simulink model "PID_Position_Control"  (R2020a)
settings: Solver=VariableStepAuto  StartTime=0.0  StopTime=10  RelTol=1e-3
undefined symbols (not defined in the file or in its folder): X, Y, Z
libraries: sm_lib x79, nesl_utility x41, simulink x24
(part 2 of 3)

== system PID_Position_Control/PID Control/C9 ==
  Radian : Inport
  Expect : Inport  Port=2
  Discrete Derivative : simulink/Discrete/Discrete Derivative  gainval=1.0  ICPrevScaledInput=0.0  OutMin=[]  OutMax=[]  OutDataType=fixdt(1, 16)  OutScaling=2^-10  DoSatur=off
  Discrete PID Controller : simulink/Continuous/PID Controller  Controller=PID  Form=Parallel  TimeDomain=Discrete-time  UseExternalTs=off  SampleTime=-1  IntegratorMethod=Forward Euler  FilterMethod=Forward Euler  ControllerParametersSource=internal  P=65  I=0.5  D=0.1  UseFilter=on  N=100  TunerSelectOption=Transfer Function Based (PID Tuner App)  InitialConditionSource=internal  InitialConditionForIntegrator=0  InitialConditionForFilter=0  DifferentiatorICPrevScaledInput=0  ExternalReset=none  TrackingMode=off  Kt=1  LimitOutput=off  UpperSaturationLimit=inf  LowerSaturationLimit=-inf  LinearizeAsGain=off  AntiWindupMode=none  Kb=1  POutMin=[]  POutMax=[]  IOutMin=[]  IOutMax=[]  DOutMin=[]  DOutMax=[]  NOutMin=[]  NOutMax=[]  SumOutMin=[]  SumOutMax=[]  SaturationOutMin=[]  SaturationOutMax=[]  PParamMin=[]  PParamMax=[]  IParamMin=[]  IParamMax=[]  DParamMin=[]  DParamMax=[]  NParamMin=[]  NParamMax=[]  KbParamMin=[]  KbParamMax=[]  KtParamMin=[]  KtParamMax=[]  KbOutMin=[]  KbOutMax=[]  KtOutMin=[]  KtOutMax=[]  IntegratorOutMin=[]  IntegratorOutMax=[]  FilterOutMin=[]  FilterOutMax=[]  SumI1OutMin=[]  SumI1OutMax=[]  SumI2OutMin=[]  SumI2OutMax=[]  SumI3OutMin=[]  SumI3OutMax=[]  SumI4OutMin=[]  SumI4OutMax=[]  SumDOutMin=[]  SumDOutMax=[]  DifferentiatorOutMin=[]  DifferentiatorOutMax=[]  FilterDiffOutCoefMin=[]  FilterDiffOutCoefMax=[]  ReciprocalOutMin=[]  ReciprocalOutMax=[]  SumDenOutMin=[]  SumDenOutMax=[]  SumNumOutMin=[]  SumNumOutMax=[]  DivideOutMin=[]  DivideOutMax=[]  UdiffTsProdOutMin=[]  UdiffTsProdOutMax=[]  NTsProdOutMin=[]  NTsProdOutMax=[]  UintegralTsProdOutMin=[]  UintegralTsProdOutMax=[]  UngainTsProdOutMin=[]  UngainTsProdOutMax=[]  IntegratorContinuousStateAttributes=''  IntegratorStateMustResolveToSignalObject=off  IntegratorRTWStateStorageClass=Auto  FilterContinuousStateAttributes=''  FilterStateMustResolveToSignalObject=off  FilterRTWStateStorageClass=Auto  ParallelPVariant=InternalParameters  IdealPVariant=Disabled  IVariant=InternalParameters  DVariant=InternalParameters  IntegratorVariant=Discrete  SatVariant=Disabled  AWVariant=Passthrough  PCopyVariant=Disabled  TRVariant=Disabled  FdbkBlocksVariant=Forward  IdealPFdbkVariant=Disabled  SatFdbkVariant=Disabled  DerivativeFilterVariant=ForwardEulerFilter  NVariant=InternalParameters  NCopyVariant=Disabled  FilterICVariant=InternalICsFilter  IntegratorICVariant=InternalICs  ExternalResetVariant=Disabled  TRSumVariant=Passthrough  SumFdbkVariant=Disabled  SumVariant=Sum_PID  TsampFilterVariant=InternalTs  TsampNgainVariant=Passthrough  TsampIntegralVariant=Passthrough
  Discrete PID Controller1 : simulink/Continuous/PID Controller  Controller=PID  Form=Parallel  TimeDomain=Discrete-time  UseExternalTs=off  SampleTime=-1  IntegratorMethod=Forward Euler  FilterMethod=Forward Euler  ControllerParametersSource=internal  P=27  I=15  D=0.1  UseFilter=on  N=100  TunerSelectOption=Transfer Function Based (PID Tuner App)  InitialConditionSource=internal  InitialConditionForIntegrator=0  InitialConditionForFilter=0  DifferentiatorICPrevScaledInput=0  ExternalReset=none  TrackingMode=off  Kt=1  LimitOutput=off  UpperSaturationLimit=inf  LowerSaturationLimit=-inf  LinearizeAsGain=off  AntiWindupMode=none  Kb=1  POutMin=[]  POutMax=[]  IOutMin=[]  IOutMax=[]  DOutMin=[]  DOutMax=[]  NOutMin=[]  NOutMax=[]  SumOutMin=[]  SumOutMax=[]  SaturationOutMin=[]  SaturationOutMax=[]  PParamMin=[]  PParamMax=[]  IParamMin=[]  IParamMax=[]  DParamMin=[]  DParamMax=[]  NParamMin=[]  NParamMax=[]  KbParamMin=[]  KbParamMax=[]  KtParamMin=[]  KtParamMax=[]  KbOutMin=[]  KbOutMax=[]  KtOutMin=[]  KtOutMax=[]  IntegratorOutMin=[]  IntegratorOutMax=[]  FilterOutMin=[]  FilterOutMax=[]  SumI1OutMin=[]  SumI1OutMax=[]  SumI2OutMin=[]  SumI2OutMax=[]  SumI3OutMin=[]  SumI3OutMax=[]  SumI4OutMin=[]  SumI4OutMax=[]  SumDOutMin=[]  SumDOutMax=[]  DifferentiatorOutMin=[]  DifferentiatorOutMax=[]  FilterDiffOutCoefMin=[]  FilterDiffOutCoefMax=[]  ReciprocalOutMin=[]  ReciprocalOutMax=[]  SumDenOutMin=[]  SumDenOutMax=[]  SumNumOutMin=[]  SumNumOutMax=[]  DivideOutMin=[]  DivideOutMax=[]  UdiffTsProdOutMin=[]  UdiffTsProdOutMax=[]  NTsProdOutMin=[]  NTsProdOutMax=[]  UintegralTsProdOutMin=[]  UintegralTsProdOutMax=[]  UngainTsProdOutMin=[]  UngainTsProdOutMax=[]  IntegratorContinuousStateAttributes=''  IntegratorStateMustResolveToSignalObject=off  IntegratorRTWStateStorageClass=Auto  FilterContinuousStateAttributes=''  FilterStateMustResolveToSignalObject=off  FilterRTWStateStorageClass=Auto  ParallelPVariant=InternalParameters  IdealPVariant=Disabled  IVariant=InternalParameters  DVariant=InternalParameters  IntegratorVariant=Discrete  SatVariant=Disabled  AWVariant=Passthrough  PCopyVariant=Disabled  TRVariant=Disabled  FdbkBlocksVariant=Forward  IdealPFdbkVariant=Disabled  SatFdbkVariant=Disabled  DerivativeFilterVariant=ForwardEulerFilter  NVariant=InternalParameters  NCopyVariant=Disabled  FilterICVariant=InternalICsFilter  IntegratorICVariant=InternalICs  ExternalResetVariant=Disabled  TRSumVariant=Passthrough  SumFdbkVariant=Disabled  SumVariant=Sum_PID  TsampFilterVariant=InternalTs  TsampNgainVariant=Passthrough  TsampIntegralVariant=Passthrough
  Sum : Sum  Inputs=|+-
  Sum1 : Sum  Inputs=|+-
  Tau : Outport  VectorParamsAs1DForOutWhenUnconnected=off
  wires:
  Discrete PID Controller1/1 -> Tau/1
  Sum/1 -> Discrete PID Controller/1
  Radian/1 -> Discrete Derivative/1, Sum/2
  Expect/1 -> Sum/1
  Discrete Derivative/1 -> Sum1/2
  Discrete PID Controller/1 -> Sum1/1
  Sum1/1 -> Discrete PID Controller1/1

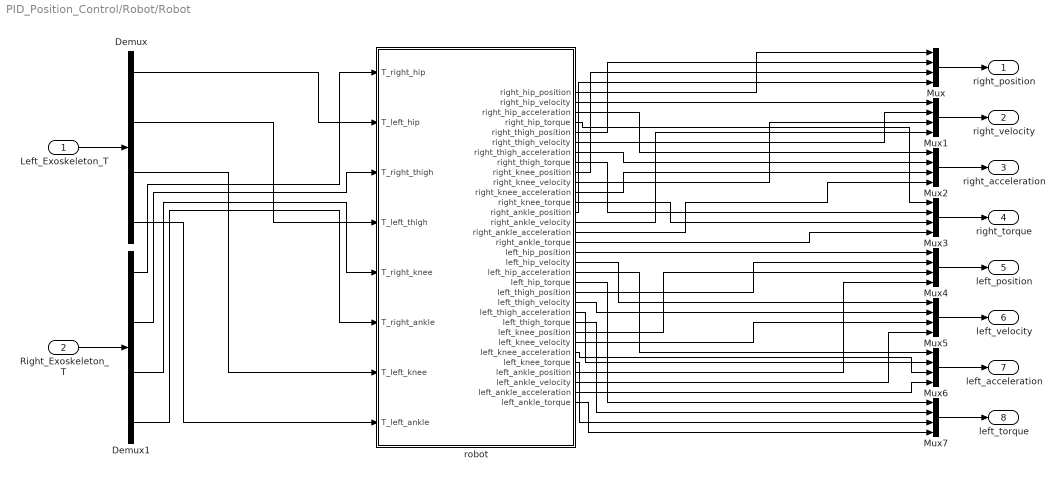
== system PID_Position_Control/Robot/Robot ==
  Left_Exoskeleton_T : Inport
  Right_Exoskeleton_T : Inport  Port=2
  Demux : Demux
  Demux1 : Demux
  Mux{,1..7} (8 alike) : Mux
  robot : Subsystem
  right_position : Outport  VectorParamsAs1DForOutWhenUnconnected=off
  right_velocity : Outport  Port=2  VectorParamsAs1DForOutWhenUnconnected=off
  right_acceleration : Outport  Port=3  VectorParamsAs1DForOutWhenUnconnected=off
  right_torque : Outport  Port=4  VectorParamsAs1DForOutWhenUnconnected=off
  left_position : Outport  Port=5  VectorParamsAs1DForOutWhenUnconnected=off
  left_velocity : Outport  Port=6  VectorParamsAs1DForOutWhenUnconnected=off
  left_acceleration : Outport  Port=7  VectorParamsAs1DForOutWhenUnconnected=off
  left_torque : Outport  Port=8  VectorParamsAs1DForOutWhenUnconnected=off
  wires:
  Demux/1 -> robot/2(T_left_hip)
  robot/14(right_ankle_velocity) -> Mux1/4
  Left_Exoskeleton_T/1 -> Demux/1
  robot/12(right_knee_torque) -> Mux3/3
  robot/31(left_ankle_acceleration) -> Mux6/4
  Demux1/4 -> robot/6(T_right_ankle)
  robot/17(left_hip_position) -> Mux4/1
  robot/22(left_thigh_velocity) -> Mux5/2
  robot/27(left_knee_acceleration) -> Mux6/3
  Mux/1 -> right_position/1
  Mux7/1 -> left_torque/1
  robot/5(right_thigh_position) -> Mux/2
  robot/16(right_ankle_torque) -> Mux3/4
  robot/3(right_hip_acceleration) -> Mux2/1
  robot/18(left_hip_velocity) -> Mux5/1
  Demux1/1 -> robot/1(T_right_hip)
  Demux1/3 -> robot/5(T_right_knee)
  robot/8(right_thigh_torque) -> Mux3/2
  robot/10(right_knee_velocity) -> Mux1/3
  Demux/4 -> robot/8(T_left_ankle)
  robot/24(left_thigh_torque) -> Mux7/2
  Mux3/1 -> right_torque/1
  robot/15(right_ankle_acceleration) -> Mux2/4
  robot/7(right_thigh_acceleration) -> Mux2/2
  robot/21(left_thigh_position) -> Mux4/2
  robot/4(right_hip_torque) -> Mux3/1
  Mux1/1 -> right_velocity/1
  robot/1(right_hip_position) -> Mux/1
  robot/29(left_ankle_position) -> Mux4/4
  robot/20(left_hip_torque) -> Mux7/1
  Mux4/1 -> left_position/1
  robot/25(left_knee_position) -> Mux4/3
  robot/9(right_knee_position) -> Mux/3
  robot/32(left_ankle_torque) -> Mux7/4
  Mux2/1 -> right_acceleration/1
  robot/19(left_hip_acceleration) -> Mux6/1
  Mux5/1 -> left_velocity/1
  robot/11(right_knee_acceleration) -> Mux2/3
  robot/26(left_knee_velocity) -> Mux5/3
  robot/13(right_ankle_position) -> Mux/4
  robot/2(right_hip_velocity) -> Mux1/1
  robot/28(left_knee_torque) -> Mux7/3
  robot/30(left_ankle_velocity) -> Mux5/4
  Mux6/1 -> left_acceleration/1
  Demux/3 -> robot/7(T_left_knee)
  Demux1/2 -> robot/3(T_right_thigh)
  Right_Exoskeleton_T/1 -> Demux1/1
  Demux/2 -> robot/4(T_left_thigh)
  robot/6(right_thigh_velocity) -> Mux1/2
  robot/23(left_thigh_acceleration) -> Mux6/2

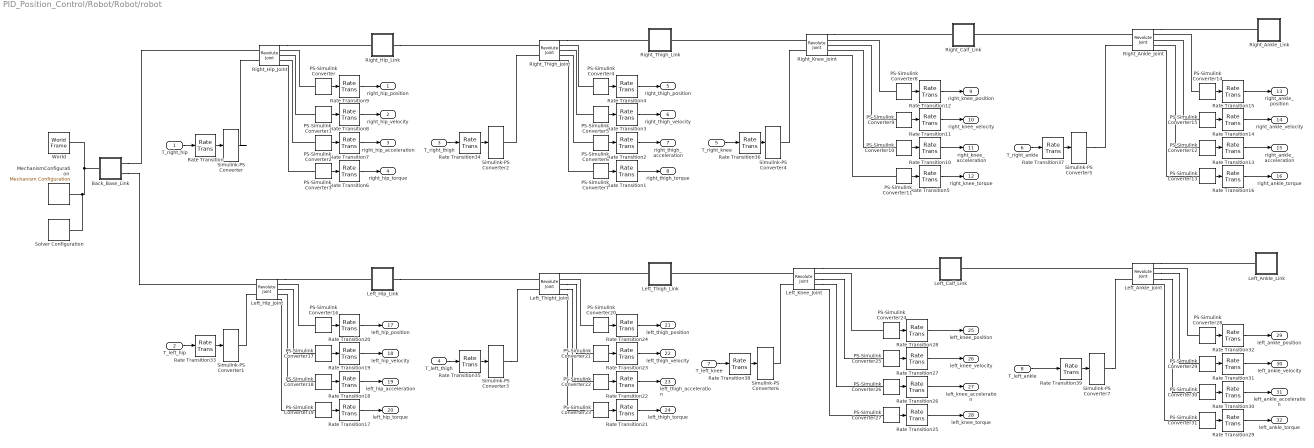
== system PID_Position_Control/Robot/Robot/robot ==
  T_right_hip : Inport
  T_left_hip : Inport  Port=2
  T_right_thigh : Inport  Port=3
  T_left_thigh : Inport  Port=4
  T_right_knee : Inport  Port=5
  T_right_ankle : Inport  Port=6
  T_left_knee : Inport  Port=7
  T_left_ankle : Inport  Port=8
  Back_Base_Link : Subsystem
  Left_Ankle_Joint : sm_lib/Joints/Revolute Joint  JointMode=Normal  SenseConstraintForce=off  SenseConstraintForceX=off  SenseConstraintForceY=off  SenseConstraintForceZ=off  SenseConstraintTorque=off  SenseConstraintTorqueX=off  SenseConstraintTorqueY=off  SenseConstraintTorqueZ=off  SenseTotalForce=off  SenseTotalForceX=off  SenseTotalForceY=off  SenseTotalForceZ=off  SenseTotalTorque=off  SenseTotalTorqueX=off  SenseTotalTorqueY=off  SenseTotalTorqueZ=off  CompositeWrenchDir=FollowerOnBase  CompositeWrenchFrame=BaseFrame  EquilibriumPosition=0  EquilibriumPositionUnits=deg  SpringStiffness=0  SpringStiffnessUnits=N*m/deg  DampingCoefficient=0  DampingCoefficientUnits=m^2*kg/s/rad  TorqueActuationMode=InputTorque  MotionActuationMode=ComputedMotion  SensePosition=on  SenseVelocity=on  SenseAcceleration=on  SenseTorqueForce=on  SenseLowerLimitTorqueForce=off  SenseUpperLimitTorqueForce=off  LowerLimitSpecify=off  LowerLimitBound=0  LowerLimitBoundUnits=rad  LowerLimitStiffness=1e4  LowerLimitStiffnessUnits=N*m/deg  LowerLimitDamping=10  LowerLimitDampingUnits=N*m/(deg/s)  LowerLimitTransitionRegionWidth=0.1  LowerLimitTransitionRegionWidthUnits=deg  UpperLimitSpecify=off  UpperLimitBound=0  UpperLimitBoundUnits=rad  UpperLimitStiffness=1e4  UpperLimitStiffnessUnits=N*m/deg  UpperLimitDamping=10  UpperLimitDampingUnits=N*m/(deg/s)  UpperLimitTransitionRegionWidth=0.1  UpperLimitTransitionRegionWidthUnits=deg  PositionTargetSpecify=off  PositionTargetPriority=High  PositionTargetValue=0  PositionTargetValueUnits=deg  VelocityTargetSpecify=off  VelocityTargetPriority=High  VelocityTargetValue=0  VelocityTargetValueUnits=deg/s
  Left_Ankle_Link : Subsystem
  Left_Calf_Link : Subsystem
  Left_Hip_Joint : sm_lib/Joints/Revolute Joint  JointMode=Normal  SenseConstraintForce=off  SenseConstraintForceX=off  SenseConstraintForceY=off  SenseConstraintForceZ=off  SenseConstraintTorque=off  SenseConstraintTorqueX=off  SenseConstraintTorqueY=off  SenseConstraintTorqueZ=off  SenseTotalForce=off  SenseTotalForceX=off  SenseTotalForceY=off  SenseTotalForceZ=off  SenseTotalTorque=off  SenseTotalTorqueX=off  SenseTotalTorqueY=off  SenseTotalTorqueZ=off  CompositeWrenchDir=FollowerOnBase  CompositeWrenchFrame=BaseFrame  EquilibriumPosition=0  EquilibriumPositionUnits=deg  SpringStiffness=0  SpringStiffnessUnits=N*m/deg  DampingCoefficient=0  DampingCoefficientUnits=m^2*kg/s/rad  TorqueActuationMode=InputTorque  MotionActuationMode=ComputedMotion  SensePosition=on  SenseVelocity=on  SenseAcceleration=on  SenseTorqueForce=on  SenseLowerLimitTorqueForce=off  SenseUpperLimitTorqueForce=off  LowerLimitSpecify=off  LowerLimitBound=0  LowerLimitBoundUnits=rad  LowerLimitStiffness=1e4  LowerLimitStiffnessUnits=N*m/deg  LowerLimitDamping=10  LowerLimitDampingUnits=N*m/(deg/s)  LowerLimitTransitionRegionWidth=0.1  LowerLimitTransitionRegionWidthUnits=deg  UpperLimitSpecify=off  UpperLimitBound=0  UpperLimitBoundUnits=rad  UpperLimitStiffness=1e4  UpperLimitStiffnessUnits=N*m/deg  UpperLimitDamping=10  UpperLimitDampingUnits=N*m/(deg/s)  UpperLimitTransitionRegionWidth=0.1  UpperLimitTransitionRegionWidthUnits=deg  PositionTargetSpecify=off  PositionTargetPriority=High  PositionTargetValue=0  PositionTargetValueUnits=deg  VelocityTargetSpecify=off  VelocityTargetPriority=High  VelocityTargetValue=0  VelocityTargetValueUnits=deg/s
  Left_Hip_Link : Subsystem
  Left_Knee_Joint : sm_lib/Joints/Revolute Joint  JointMode=Normal  SenseConstraintForce=off  SenseConstraintForceX=off  SenseConstraintForceY=off  SenseConstraintForceZ=off  SenseConstraintTorque=off  SenseConstraintTorqueX=off  SenseConstraintTorqueY=off  SenseConstraintTorqueZ=off  SenseTotalForce=off  SenseTotalForceX=off  SenseTotalForceY=off  SenseTotalForceZ=off  SenseTotalTorque=off  SenseTotalTorqueX=off  SenseTotalTorqueY=off  SenseTotalTorqueZ=off  CompositeWrenchDir=FollowerOnBase  CompositeWrenchFrame=BaseFrame  EquilibriumPosition=0  EquilibriumPositionUnits=deg  SpringStiffness=0  SpringStiffnessUnits=N*m/deg  DampingCoefficient=0  DampingCoefficientUnits=m^2*kg/s/rad  TorqueActuationMode=InputTorque  MotionActuationMode=ComputedMotion  SensePosition=on  SenseVelocity=on  SenseAcceleration=on  SenseTorqueForce=on  SenseLowerLimitTorqueForce=off  SenseUpperLimitTorqueForce=off  LowerLimitSpecify=off  LowerLimitBound=0  LowerLimitBoundUnits=rad  LowerLimitStiffness=1e4  LowerLimitStiffnessUnits=N*m/deg  LowerLimitDamping=10  LowerLimitDampingUnits=N*m/(deg/s)  LowerLimitTransitionRegionWidth=0.1  LowerLimitTransitionRegionWidthUnits=deg  UpperLimitSpecify=off  UpperLimitBound=0  UpperLimitBoundUnits=rad  UpperLimitStiffness=1e4  UpperLimitStiffnessUnits=N*m/deg  UpperLimitDamping=10  UpperLimitDampingUnits=N*m/(deg/s)  UpperLimitTransitionRegionWidth=0.1  UpperLimitTransitionRegionWidthUnits=deg  PositionTargetSpecify=off  PositionTargetPriority=High  PositionTargetValue=0  PositionTargetValueUnits=deg  VelocityTargetSpecify=off  VelocityTargetPriority=High  VelocityTargetValue=0  VelocityTargetValueUnits=deg/s
  Left_Thigh_Link : Subsystem
  Left_Thight_Joint : sm_lib/Joints/Revolute Joint  JointMode=Normal  SenseConstraintForce=off  SenseConstraintForceX=off  SenseConstraintForceY=off  SenseConstraintForceZ=off  SenseConstraintTorque=off  SenseConstraintTorqueX=off  SenseConstraintTorqueY=off  SenseConstraintTorqueZ=off  SenseTotalForce=off  SenseTotalForceX=off  SenseTotalForceY=off  SenseTotalForceZ=off  SenseTotalTorque=off  SenseTotalTorqueX=off  SenseTotalTorqueY=off  SenseTotalTorqueZ=off  CompositeWrenchDir=FollowerOnBase  CompositeWrenchFrame=BaseFrame  EquilibriumPosition=0  EquilibriumPositionUnits=deg  SpringStiffness=0  SpringStiffnessUnits=N*m/deg  DampingCoefficient=0  DampingCoefficientUnits=m^2*kg/s/rad  TorqueActuationMode=InputTorque  MotionActuationMode=ComputedMotion  SensePosition=on  SenseVelocity=on  SenseAcceleration=on  SenseTorqueForce=on  SenseLowerLimitTorqueForce=off  SenseUpperLimitTorqueForce=off  LowerLimitSpecify=off  LowerLimitBound=0  LowerLimitBoundUnits=rad  LowerLimitStiffness=1e4  LowerLimitStiffnessUnits=N*m/deg  LowerLimitDamping=10  LowerLimitDampingUnits=N*m/(deg/s)  LowerLimitTransitionRegionWidth=0.1  LowerLimitTransitionRegionWidthUnits=deg  UpperLimitSpecify=off  UpperLimitBound=0  UpperLimitBoundUnits=rad  UpperLimitStiffness=1e4  UpperLimitStiffnessUnits=N*m/deg  UpperLimitDamping=10  UpperLimitDampingUnits=N*m/(deg/s)  UpperLimitTransitionRegionWidth=0.1  UpperLimitTransitionRegionWidthUnits=deg  PositionTargetSpecify=off  PositionTargetPriority=High  PositionTargetValue=0  PositionTargetValueUnits=deg  VelocityTargetSpecify=off  VelocityTargetPriority=High  VelocityTargetValue=0  VelocityTargetValueUnits=deg/s
  MechanismConfiguration : sm_lib/Utilities/Mechanism Configuration  UniformGravity=Constant  GravityVector=[0 0 -9.80665]  GravityUnits=m/s^2  LinearizationDelta=0.001
  PS-Simulink Converter{,4,8,14,16,20,24,28} (8 alike) : nesl_utility/PS-Simulink Converter  PhysicalDomain=network_engine_domain  SubClassName=ps_output  LeftPortType=input  RightPortType=output  PseudoPeriodic=off  Frequencies=[]  Unit=rad  AffineConversion=off
  PS-Simulink Converter{1,5,9,15,17,21,25,29} (8 alike) : nesl_utility/PS-Simulink Converter  PhysicalDomain=network_engine_domain  SubClassName=ps_output  LeftPortType=input  RightPortType=output  PseudoPeriodic=off  Frequencies=[]  Unit=rad/s  AffineConversion=off
  PS-Simulink Converter{2,6,10,12,18,22,26,30} (8 alike) : nesl_utility/PS-Simulink Converter  PhysicalDomain=network_engine_domain  SubClassName=ps_output  LeftPortType=input  RightPortType=output  PseudoPeriodic=off  Frequencies=[]  Unit=1  AffineConversion=off
  PS-Simulink Converter{3,7,11,13,19,23,27,31} (8 alike) : nesl_utility/PS-Simulink Converter  PhysicalDomain=network_engine_domain  SubClassName=ps_output  LeftPortType=input  RightPortType=output  PseudoPeriodic=off  Frequencies=[]  Unit=N*m  AffineConversion=off
  Rate Transition{,1..39} (40 alike) : RateTransition
  Right_Ankle_Joint : sm_lib/Joints/Revolute Joint  JointMode=Normal  SenseConstraintForce=off  SenseConstraintForceX=off  SenseConstraintForceY=off  SenseConstraintForceZ=off  SenseConstraintTorque=off  SenseConstraintTorqueX=off  SenseConstraintTorqueY=off  SenseConstraintTorqueZ=off  SenseTotalForce=off  SenseTotalForceX=off  SenseTotalForceY=off  SenseTotalForceZ=off  SenseTotalTorque=off  SenseTotalTorqueX=off  SenseTotalTorqueY=off  SenseTotalTorqueZ=off  CompositeWrenchDir=FollowerOnBase  CompositeWrenchFrame=BaseFrame  EquilibriumPosition=0  EquilibriumPositionUnits=deg  SpringStiffness=0  SpringStiffnessUnits=N*m/deg  DampingCoefficient=0  DampingCoefficientUnits=m^2*kg/s/rad  TorqueActuationMode=InputTorque  MotionActuationMode=ComputedMotion  SensePosition=on  SenseVelocity=on  SenseAcceleration=on  SenseTorqueForce=on  SenseLowerLimitTorqueForce=off  SenseUpperLimitTorqueForce=off  LowerLimitSpecify=off  LowerLimitBound=0  LowerLimitBoundUnits=rad  LowerLimitStiffness=1e4  LowerLimitStiffnessUnits=N*m/deg  LowerLimitDamping=10  LowerLimitDampingUnits=N*m/(deg/s)  LowerLimitTransitionRegionWidth=0.1  LowerLimitTransitionRegionWidthUnits=deg  UpperLimitSpecify=off  UpperLimitBound=0  UpperLimitBoundUnits=rad  UpperLimitStiffness=1e4  UpperLimitStiffnessUnits=N*m/deg  UpperLimitDamping=10  UpperLimitDampingUnits=N*m/(deg/s)  UpperLimitTransitionRegionWidth=0.1  UpperLimitTransitionRegionWidthUnits=deg  PositionTargetSpecify=off  PositionTargetPriority=High  PositionTargetValue=0  PositionTargetValueUnits=deg  VelocityTargetSpecify=off  VelocityTargetPriority=High  VelocityTargetValue=0  VelocityTargetValueUnits=deg/s
  Right_Ankle_Link : Subsystem
  Right_Calf_Link : Subsystem
  Right_Hip_Joint : sm_lib/Joints/Revolute Joint  JointMode=Normal  SenseConstraintForce=off  SenseConstraintForceX=off  SenseConstraintForceY=off  SenseConstraintForceZ=off  SenseConstraintTorque=off  SenseConstraintTorqueX=off  SenseConstraintTorqueY=off  SenseConstraintTorqueZ=off  SenseTotalForce=off  SenseTotalForceX=off  SenseTotalForceY=off  SenseTotalForceZ=off  SenseTotalTorque=off  SenseTotalTorqueX=off  SenseTotalTorqueY=off  SenseTotalTorqueZ=off  CompositeWrenchDir=FollowerOnBase  CompositeWrenchFrame=BaseFrame  EquilibriumPosition=0  EquilibriumPositionUnits=deg  SpringStiffness=0  SpringStiffnessUnits=N*m/deg  DampingCoefficient=0  DampingCoefficientUnits=m^2*kg/s/rad  TorqueActuationMode=InputTorque  MotionActuationMode=ComputedMotion  SensePosition=on  SenseVelocity=on  SenseAcceleration=on  SenseTorqueForce=on  SenseLowerLimitTorqueForce=off  SenseUpperLimitTorqueForce=off  LowerLimitSpecify=off  LowerLimitBound=0  LowerLimitBoundUnits=rad  LowerLimitStiffness=1e4  LowerLimitStiffnessUnits=N*m/deg  LowerLimitDamping=10  LowerLimitDampingUnits=N*m/(deg/s)  LowerLimitTransitionRegionWidth=0.1  LowerLimitTransitionRegionWidthUnits=deg  UpperLimitSpecify=off  UpperLimitBound=0  UpperLimitBoundUnits=rad  UpperLimitStiffness=1e4  UpperLimitStiffnessUnits=N*m/deg  UpperLimitDamping=10  UpperLimitDampingUnits=N*m/(deg/s)  UpperLimitTransitionRegionWidth=0.1  UpperLimitTransitionRegionWidthUnits=deg  PositionTargetSpecify=off  PositionTargetPriority=High  PositionTargetValue=0  PositionTargetValueUnits=deg  VelocityTargetSpecify=off  VelocityTargetPriority=High  VelocityTargetValue=0  VelocityTargetValueUnits=deg/s
  Right_Hip_Link : Subsystem
  Right_Knee_Joint : sm_lib/Joints/Revolute Joint  JointMode=Normal  SenseConstraintForce=off  SenseConstraintForceX=off  SenseConstraintForceY=off  SenseConstraintForceZ=off  SenseConstraintTorque=off  SenseConstraintTorqueX=off  SenseConstraintTorqueY=off  SenseConstraintTorqueZ=off  SenseTotalForce=off  SenseTotalForceX=off  SenseTotalForceY=off  SenseTotalForceZ=off  SenseTotalTorque=off  SenseTotalTorqueX=off  SenseTotalTorqueY=off  SenseTotalTorqueZ=off  CompositeWrenchDir=FollowerOnBase  CompositeWrenchFrame=BaseFrame  EquilibriumPosition=0  EquilibriumPositionUnits=deg  SpringStiffness=0  SpringStiffnessUnits=N*m/deg  DampingCoefficient=0  DampingCoefficientUnits=m^2*kg/s/rad  TorqueActuationMode=InputTorque  MotionActuationMode=ComputedMotion  SensePosition=on  SenseVelocity=on  SenseAcceleration=on  SenseTorqueForce=on  SenseLowerLimitTorqueForce=off  SenseUpperLimitTorqueForce=off  LowerLimitSpecify=off  LowerLimitBound=0  LowerLimitBoundUnits=rad  LowerLimitStiffness=1e4  LowerLimitStiffnessUnits=N*m/deg  LowerLimitDamping=10  LowerLimitDampingUnits=N*m/(deg/s)  LowerLimitTransitionRegionWidth=0.1  LowerLimitTransitionRegionWidthUnits=deg  UpperLimitSpecify=off  UpperLimitBound=0  UpperLimitBoundUnits=rad  UpperLimitStiffness=1e4  UpperLimitStiffnessUnits=N*m/deg  UpperLimitDamping=10  UpperLimitDampingUnits=N*m/(deg/s)  UpperLimitTransitionRegionWidth=0.1  UpperLimitTransitionRegionWidthUnits=deg  PositionTargetSpecify=off  PositionTargetPriority=High  PositionTargetValue=0  PositionTargetValueUnits=deg  VelocityTargetSpecify=off  VelocityTargetPriority=High  VelocityTargetValue=0  VelocityTargetValueUnits=deg/s
  Right_Thigh_Joint : sm_lib/Joints/Revolute Joint  JointMode=Normal  SenseConstraintForce=off  SenseConstraintForceX=off  SenseConstraintForceY=off  SenseConstraintForceZ=off  SenseConstraintTorque=off  SenseConstraintTorqueX=off  SenseConstraintTorqueY=off  SenseConstraintTorqueZ=off  SenseTotalForce=off  SenseTotalForceX=off  SenseTotalForceY=off  SenseTotalForceZ=off  SenseTotalTorque=off  SenseTotalTorqueX=off  SenseTotalTorqueY=off  SenseTotalTorqueZ=off  CompositeWrenchDir=FollowerOnBase  CompositeWrenchFrame=BaseFrame  EquilibriumPosition=0  EquilibriumPositionUnits=deg  SpringStiffness=0  SpringStiffnessUnits=N*m/deg  DampingCoefficient=0  DampingCoefficientUnits=m^2*kg/s/rad  TorqueActuationMode=InputTorque  MotionActuationMode=ComputedMotion  SensePosition=on  SenseVelocity=on  SenseAcceleration=on  SenseTorqueForce=on  SenseLowerLimitTorqueForce=off  SenseUpperLimitTorqueForce=off  LowerLimitSpecify=off  LowerLimitBound=0  LowerLimitBoundUnits=rad  LowerLimitStiffness=1e4  LowerLimitStiffnessUnits=N*m/deg  LowerLimitDamping=10  LowerLimitDampingUnits=N*m/(deg/s)  LowerLimitTransitionRegionWidth=0.1  LowerLimitTransitionRegionWidthUnits=deg  UpperLimitSpecify=off  UpperLimitBound=0  UpperLimitBoundUnits=rad  UpperLimitStiffness=1e4  UpperLimitStiffnessUnits=N*m/deg  UpperLimitDamping=10  UpperLimitDampingUnits=N*m/(deg/s)  UpperLimitTransitionRegionWidth=0.1  UpperLimitTransitionRegionWidthUnits=deg  PositionTargetSpecify=off  PositionTargetPriority=High  PositionTargetValue=0  PositionTargetValueUnits=deg  VelocityTargetSpecify=off  VelocityTargetPriority=High  VelocityTargetValue=0  VelocityTargetValueUnits=deg/s
  Right_Thigh_Link : Subsystem
  Simulink-PS Converter{,1..7} (8 alike) : nesl_utility/Simulink-PS Converter  PhysicalDomain=network_engine_domain  SubClassName=ps_input  LeftPortType=input  RightPortType=output  PseudoPeriodic=off  Frequencies=[]  NoiseDistribution=none  NoiseParameters=[]  Unit=N*m  AffineConversion=off  FilteringAndDerivatives=zero  SimscapeFilterOrder=1  InputFilterTimeConstant=0.001  UdotUserProvided=2
  Solver Configuration : nesl_utility/Solver Configuration  PhysicalDomain=network_engine_domain  SubClassName=solver  LeftPortType=input  RightPortType=generic  Tones=[]  Harmonics=[]  SimulateNoise=off  Profile=off  UseLocalSampling=off  EnableSwitchedLinearOptims=on  FrequencyDomain=off  UseCCode=off  RelTol=0.001  AbsTol=1e-06  MinStep=1e-09  ToWorkspace=off  RevertToSquareIcSolve=off  NumHomotopyIterations=100  PhasorMode=off  PhasorModeNumHarmonics=1  DoDC=off  ResidualTolerance=1e-09  UseLocalSolver=off  LocalSolverChoice=NE_BACKWARD_EULER_ADVANCER  LocalSolverSampleTime=0.001  DoFixedCost=off  MaxNonlinIter=3  MaxModeIter=2  LinearAlgebra=auto  EquationFormulation=NE_TIME_EF  DelaysMemoryBudget=1024  AutomaticFiltering=on  FilteringTimeConstant=0.001  PartitionStorageMethod=AS_NEEDED  PartitionMemoryBudget=1024  PartitionMethod=ROBUST
  World : sm_lib/Frames and Transforms/World Frame
  right_hip_position : Outport  VectorParamsAs1DForOutWhenUnconnected=off
  right_hip_velocity : Outport  Port=2  VectorParamsAs1DForOutWhenUnconnected=off
  right_hip_acceleration : Outport  Port=3  VectorParamsAs1DForOutWhenUnconnected=off
  right_hip_torque : Outport  Port=4  VectorParamsAs1DForOutWhenUnconnected=off
  right_thigh_position : Outport  Port=5  VectorParamsAs1DForOutWhenUnconnected=off
  right_thigh_velocity : Outport  Port=6  VectorParamsAs1DForOutWhenUnconnected=off
  right_thigh_acceleration : Outport  Port=7  VectorParamsAs1DForOutWhenUnconnected=off
  right_thigh_torque : Outport  Port=8  VectorParamsAs1DForOutWhenUnconnected=off
  right_knee_position : Outport  Port=9  VectorParamsAs1DForOutWhenUnconnected=off
  right_knee_velocity : Outport  Port=10  VectorParamsAs1DForOutWhenUnconnected=off
  right_knee_acceleration : Outport  Port=11  VectorParamsAs1DForOutWhenUnconnected=off
  right_knee_torque : Outport  Port=12  VectorParamsAs1DForOutWhenUnconnected=off
  right_ankle_position : Outport  Port=13  VectorParamsAs1DForOutWhenUnconnected=off
  right_ankle_velocity : Outport  Port=14  VectorParamsAs1DForOutWhenUnconnected=off
  right_ankle_acceleration : Outport  Port=15  VectorParamsAs1DForOutWhenUnconnected=off
  right_ankle_torque : Outport  Port=16  VectorParamsAs1DForOutWhenUnconnected=off
  left_hip_position : Outport  Port=17  VectorParamsAs1DForOutWhenUnconnected=off
  left_hip_velocity : Outport  Port=18  VectorParamsAs1DForOutWhenUnconnected=off
  left_hip_acceleration : Outport  Port=19  VectorParamsAs1DForOutWhenUnconnected=off
  left_hip_torque : Outport  Port=20  VectorParamsAs1DForOutWhenUnconnected=off
  left_thigh_position : Outport  Port=21  VectorParamsAs1DForOutWhenUnconnected=off
  left_thigh_velocity : Outport  Port=22  VectorParamsAs1DForOutWhenUnconnected=off
  left_thigh_acceleration : Outport  Port=23  VectorParamsAs1DForOutWhenUnconnected=off
  left_thigh_torque : Outport  Port=24  VectorParamsAs1DForOutWhenUnconnected=off
  left_knee_position : Outport  Port=25  VectorParamsAs1DForOutWhenUnconnected=off
  left_knee_velocity : Outport  Port=26  VectorParamsAs1DForOutWhenUnconnected=off
  left_knee_acceleration : Outport  Port=27  VectorParamsAs1DForOutWhenUnconnected=off
  left_knee_torque : Outport  Port=28  VectorParamsAs1DForOutWhenUnconnected=off
  left_ankle_position : Outport  Port=29  VectorParamsAs1DForOutWhenUnconnected=off
  left_ankle_velocity : Outport  Port=30  VectorParamsAs1DForOutWhenUnconnected=off
  left_ankle_acceleration : Outport  Port=31  VectorParamsAs1DForOutWhenUnconnected=off
  left_ankle_torque : Outport  Port=32  VectorParamsAs1DForOutWhenUnconnected=off
  wires:
  PS-Simulink Converter8/1 -> Rate Transition12/1
  Rate Transition12/1 -> right_knee_position/1
  PS-Simulink Converter9/1 -> Rate Transition11/1
  Rate Transition5/1 -> right_knee_torque/1
  Rate Transition10/1 -> right_knee_acceleration/1
  PS-Simulink Converter3/1 -> Rate Transition6/1
  Rate Transition11/1 -> right_knee_velocity/1
  Rate Transition4/1 -> right_thigh_position/1
  Rate Transition3/1 -> right_thigh_velocity/1
  Rate Transition2/1 -> right_thigh_acceleration/1
  PS-Simulink Converter6/1 -> Rate Transition2/1
  PS-Simulink Converter5/1 -> Rate Transition3/1
  PS-Simulink Converter4/1 -> Rate Transition4/1
  Rate Transition1/1 -> right_thigh_torque/1
  T_right_ankle/1 -> Rate Transition37/1
  Rate Transition37/1 -> Simulink-PS Converter5/1
  Rate Transition39/1 -> Simulink-PS Converter7/1
  Rate Transition35/1 -> Simulink-PS Converter3/1
  T_left_thigh/1 -> Rate Transition35/1
  Rate Transition38/1 -> Simulink-PS Converter6/1
  T_left_knee/1 -> Rate Transition38/1
  T_right_knee/1 -> Rate Transition36/1
  T_right_thigh/1 -> Rate Transition34/1
  Rate Transition8/1 -> right_hip_velocity/1
  Rate Transition7/1 -> right_hip_acceleration/1
  Rate Transition9/1 -> right_hip_position/1
  Rate Transition36/1 -> Simulink-PS Converter4/1
  PS-Simulink Converter16/1 -> Rate Transition20/1
  PS-Simulink Converter19/1 -> Rate Transition17/1
  Rate Transition19/1 -> left_hip_velocity/1
  PS-Simulink Converter17/1 -> Rate Transition19/1
  Rate Transition20/1 -> left_hip_position/1
  Rate Transition18/1 -> left_hip_acceleration/1
  Rate Transition17/1 -> left_hip_torque/1
  T_right_hip/1 -> Rate Transition/1
  Rate Transition34/1 -> Simulink-PS Converter2/1
  PS-Simulink Converter18/1 -> Rate Transition18/1
  PS-Simulink Converter27/1 -> Rate Transition25/1
  Rate Transition25/1 -> left_knee_torque/1
  Rate Transition26/1 -> left_knee_acceleration/1
  Rate Transition28/1 -> left_knee_position/1
  PS-Simulink Converter11/1 -> Rate Transition5/1
  PS-Simulink Converter24/1 -> Rate Transition28/1
  PS-Simulink Converter25/1 -> Rate Transition27/1
  Rate Transition27/1 -> left_knee_velocity/1
  PS-Simulink Converter26/1 -> Rate Transition26/1
  Rate Transition/1 -> Simulink-PS Converter/1
  T_left_ankle/1 -> Rate Transition39/1
  PS-Simulink Converter23/1 -> Rate Transition21/1
  Rate Transition21/1 -> left_thigh_torque/1
  PS-Simulink Converter22/1 -> Rate Transition22/1
  PS-Simulink Converter21/1 -> Rate Transition23/1
  Rate Transition23/1 -> left_thigh_velocity/1
  PS-Simulink Converter1/1 -> Rate Transition8/1
  Rate Transition24/1 -> left_thigh_position/1
  PS-Simulink Converter7/1 -> Rate Transition1/1
  T_left_hip/1 -> Rate Transition33/1
  Rate Transition33/1 -> Simulink-PS Converter1/1
  PS-Simulink Converter12/1 -> Rate Transition13/1
  PS-Simulink Converter13/1 -> Rate Transition16/1
  PS-Simulink Converter2/1 -> Rate Transition7/1
  PS-Simulink Converter10/1 -> Rate Transition10/1
  PS-Simulink Converter/1 -> Rate Transition9/1
  PS-Simulink Converter15/1 -> Rate Transition14/1
  PS-Simulink Converter20/1 -> Rate Transition24/1
  Rate Transition14/1 -> right_ankle_velocity/1
  Rate Transition22/1 -> left_thigh_acceleration/1
  Rate Transition15/1 -> right_ankle_position/1
  PS-Simulink Converter30/1 -> Rate Transition30/1
  Rate Transition31/1 -> left_ankle_velocity/1
  PS-Simulink Converter29/1 -> Rate Transition31/1
  Rate Transition13/1 -> right_ankle_acceleration/1
  Rate Transition6/1 -> right_hip_torque/1
  Rate Transition29/1 -> left_ankle_torque/1
  Rate Transition32/1 -> left_ankle_position/1
  PS-Simulink Converter14/1 -> Rate Transition15/1
  Rate Transition16/1 -> right_ankle_torque/1
  PS-Simulink Converter31/1 -> Rate Transition29/1
  Rate Transition30/1 -> left_ankle_acceleration/1
  PS-Simulink Converter28/1 -> Rate Transition32/1
  connections:
  Back_Base_Link/LConn1 -- World/RConn1 -- Solver Configuration/RConn1 -- MechanismConfiguration/RConn1
  PS-Simulink Converter19/LConn1 -- Left_Hip_Joint/RConn5
  PS-Simulink Converter8/LConn1 -- Right_Knee_Joint/RConn2
  Right_Thigh_Joint/LConn2 -- Simulink-PS Converter2/RConn1
  PS-Simulink Converter10/LConn1 -- Right_Knee_Joint/RConn4
  Simulink-PS Converter7/RConn1 -- Left_Ankle_Joint/LConn2
  PS-Simulink Converter27/LConn1 -- Left_Knee_Joint/RConn5
  PS-Simulink Converter17/LConn1 -- Left_Hip_Joint/RConn3
  Right_Hip_Link/RConn1 -- Right_Thigh_Joint/LConn1
  Simulink-PS Converter5/RConn1 -- Right_Ankle_Joint/LConn2
  PS-Simulink Converter3/LConn1 -- Right_Hip_Joint/RConn5
  PS-Simulink Converter5/LConn1 -- Right_Thigh_Joint/RConn3
  Left_Ankle_Joint/RConn3 -- PS-Simulink Converter29/LConn1
  PS-Simulink Converter/LConn1 -- Right_Hip_Joint/RConn2
  PS-Simulink Converter31/LConn1 -- Left_Ankle_Joint/RConn5
  Right_Ankle_Joint/RConn1 -- Right_Ankle_Link/LConn1
  PS-Simulink Converter18/LConn1 -- Left_Hip_Joint/RConn4
  PS-Simulink Converter23/LConn1 -- Left_Thight_Joint/RConn5
  PS-Simulink Converter2/LConn1 -- Right_Hip_Joint/RConn4
  PS-Simulink Converter7/LConn1 -- Right_Thigh_Joint/RConn5
  Simulink-PS Converter1/RConn1 -- Left_Hip_Joint/LConn2
  Left_Thight_Joint/RConn3 -- PS-Simulink Converter21/LConn1
  Back_Base_Link/RConn2 -- Left_Hip_Joint/LConn1
  Left_Knee_Joint/RConn4 -- PS-Simulink Converter26/LConn1
  Back_Base_Link/RConn1 -- Right_Hip_Joint/LConn1
  PS-Simulink Converter12/LConn1 -- Right_Ankle_Joint/RConn4
  PS-Simulink Converter28/LConn1 -- Left_Ankle_Joint/RConn2
  PS-Simulink Converter14/LConn1 -- Right_Ankle_Joint/RConn2
  PS-Simulink Converter11/LConn1 -- Right_Knee_Joint/RConn5
  Left_Thight_Joint/RConn4 -- PS-Simulink Converter22/LConn1
  PS-Simulink Converter4/LConn1 -- Right_Thigh_Joint/RConn2
  Right_Knee_Joint/LConn2 -- Simulink-PS Converter4/RConn1
  Left_Knee_Joint/RConn3 -- PS-Simulink Converter25/LConn1
  Right_Hip_Joint/RConn1 -- Right_Hip_Link/LConn1
  PS-Simulink Converter16/LConn1 -- Left_Hip_Joint/RConn2
  Left_Ankle_Joint/LConn1 -- Left_Calf_Link/RConn1
  PS-Simulink Converter1/LConn1 -- Right_Hip_Joint/RConn3
  Left_Ankle_Joint/RConn1 -- Left_Ankle_Link/LConn1
  Left_Hip_Joint/RConn1 -- Left_Hip_Link/LConn1
  Left_Knee_Joint/LConn1 -- Left_Thigh_Link/RConn1
  Right_Knee_Joint/LConn1 -- Right_Thigh_Link/RConn1
  Right_Knee_Joint/RConn1 -- Right_Calf_Link/LConn1
  PS-Simulink Converter15/LConn1 -- Right_Ankle_Joint/RConn3
  Left_Hip_Link/RConn1 -- Left_Thight_Joint/LConn1
  Simulink-PS Converter3/RConn1 -- Left_Thight_Joint/LConn2
  Simulink-PS Converter/RConn1 -- Right_Hip_Joint/LConn2
  Right_Thigh_Joint/RConn1 -- Right_Thigh_Link/LConn1
  PS-Simulink Converter24/LConn1 -- Left_Knee_Joint/RConn2
  Left_Thigh_Link/LConn1 -- Left_Thight_Joint/RConn1
  PS-Simulink Converter20/LConn1 -- Left_Thight_Joint/RConn2
  Right_Ankle_Joint/LConn1 -- Right_Calf_Link/RConn1
  Left_Knee_Joint/RConn1 -- Left_Calf_Link/LConn1
  PS-Simulink Converter13/LConn1 -- Right_Ankle_Joint/RConn5
  PS-Simulink Converter9/LConn1 -- Right_Knee_Joint/RConn3
  Left_Ankle_Joint/RConn4 -- PS-Simulink Converter30/LConn1
  PS-Simulink Converter6/LConn1 -- Right_Thigh_Joint/RConn4
  Simulink-PS Converter6/RConn1 -- Left_Knee_Joint/LConn2

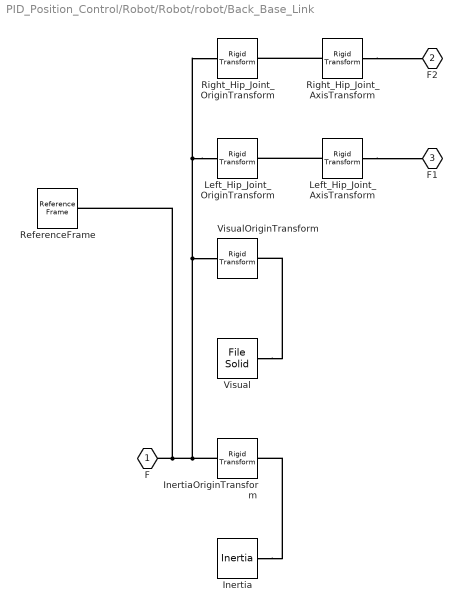
== system PID_Position_Control/Robot/Robot/robot/Back_Base_Link ==
  Inertia : sm_lib/Body Elements/Inertia  InertiaType=Custom  Mass=7.1666344893724  MassUnits=kg  CenterOfMass=[0, 0, 0]  CenterOfMassUnits=m  MomentsOfInertia=[0.287991764742564, 0.218183102338654, 0.12372998211452]  MomentsOfInertiaUnits=kg*m^2  ProductsOfInertia=[-5.72291606644722e-09, 0.00975876307734881, 4.03119244398634e-09]  ProductsOfInertiaUnits=kg*m^2  GraphicType=None  MarkerShape=Inertia  MarkerSize=20  GraphicVisPropType=SimpleVisualProperties  GraphicDiffuseColor=[0.5 0.5 0.5]  GraphicSpecularColor=[0.5 0.5 0.5 1.0]  GraphicAmbientColor=[0.15 0.15 0.15 1.0]  GraphicEmissiveColor=[0.0 0.0 0.0 1.0]  GraphicShininess=75  GraphicOpacity=1.0
  InertiaOriginTransform : sm_lib/Frames and Transforms/Rigid Transform  TranslationMethod=Cartesian  TranslationStandardOffset=0  TranslationLengthUnit=m  TranslationStandardAxis=+Z  TranslationCartesianOffset=[0.102999774541297, 1.05565171604205e-08, -0.01817224156931]  TranslationROffset=0  TranslationROffsetUnits=m  TranslationZOffset=0  TranslationZOffsetUnits=m  TranslationThetaOffset=0  TranslationThetaOffsetUnits=deg  RotationMethod=RotationSequence  RotationAngleUnits=deg  RotationStandardAxis=+Z  RotationAngle=0.0  RotationArbitraryAxis=[0 0 1]  FollAlignAxisA=+X  BaseAlignAxisA=+Y  FollAlignAxisB=+Y  BaseAlignAxisB=+Z  RotationSequenceAxes=BaseAxes  RotationSequence=XYZ  RotationSequenceAngles=[0, 0, 0]  RotationSequenceAnglesUnits=rad  RotationMatrix=[1 0 0; 0 1 0; 0 0 1]
  Left_Hip_Joint_AxisTransform : sm_lib/Frames and Transforms/Rigid Transform  TranslationMethod=Cartesian  TranslationStandardOffset=0  TranslationLengthUnit=m  TranslationStandardAxis=+Z  TranslationCartesianOffset=[0, 0, 0]  TranslationROffset=0  TranslationROffsetUnits=m  TranslationZOffset=0  TranslationZOffsetUnits=m  TranslationThetaOffset=0  TranslationThetaOffsetUnits=deg  RotationMethod=ArbitraryAxis  RotationAngleUnits=rad  RotationStandardAxis=+Z  RotationAngle=3.141592653589793  RotationArbitraryAxis=[1, 0, 0]  FollAlignAxisA=+X  BaseAlignAxisA=+Y  FollAlignAxisB=+Y  BaseAlignAxisB=+Z  RotationSequenceAxes=FollowerAxes  RotationSequence=XYX  RotationSequenceAngles=[0 0 0]  RotationSequenceAnglesUnits=deg  RotationMatrix=[1 0 0; 0 1 0; 0 0 1]
  Left_Hip_Joint_OriginTransform : sm_lib/Frames and Transforms/Rigid Transform  TranslationMethod=Cartesian  TranslationStandardOffset=0  TranslationLengthUnit=m  TranslationStandardAxis=+Z  TranslationCartesianOffset=[0.2243, 0.208, -0.283]  TranslationROffset=0  TranslationROffsetUnits=m  TranslationZOffset=0  TranslationZOffsetUnits=m  TranslationThetaOffset=0  TranslationThetaOffsetUnits=deg  RotationMethod=RotationSequence  RotationAngleUnits=deg  RotationStandardAxis=+Z  RotationAngle=0.0  RotationArbitraryAxis=[0 0 1]  FollAlignAxisA=+X  BaseAlignAxisA=+Y  FollAlignAxisB=+Y  BaseAlignAxisB=+Z  RotationSequenceAxes=BaseAxes  RotationSequence=XYZ  RotationSequenceAngles=[0, 0, 0]  RotationSequenceAnglesUnits=rad  RotationMatrix=[1 0 0; 0 1 0; 0 0 1]
  ReferenceFrame : sm_lib/Frames and Transforms/Reference Frame
  Right_Hip_Joint_AxisTransform : sm_lib/Frames and Transforms/Rigid Transform  TranslationMethod=Cartesian  TranslationStandardOffset=0  TranslationLengthUnit=m  TranslationStandardAxis=+Z  TranslationCartesianOffset=[0, 0, 0]  TranslationROffset=0  TranslationROffsetUnits=m  TranslationZOffset=0  TranslationZOffsetUnits=m  TranslationThetaOffset=0  TranslationThetaOffsetUnits=deg  RotationMethod=ArbitraryAxis  RotationAngleUnits=rad  RotationStandardAxis=+Z  RotationAngle=0  RotationArbitraryAxis=[1, 0, 0]  FollAlignAxisA=+X  BaseAlignAxisA=+Y  FollAlignAxisB=+Y  BaseAlignAxisB=+Z  RotationSequenceAxes=FollowerAxes  RotationSequence=XYX  RotationSequenceAngles=[0 0 0]  RotationSequenceAnglesUnits=deg  RotationMatrix=[1 0 0; 0 1 0; 0 0 1]
  Right_Hip_Joint_OriginTransform : sm_lib/Frames and Transforms/Rigid Transform  TranslationMethod=Cartesian  TranslationStandardOffset=0  TranslationLengthUnit=m  TranslationStandardAxis=+Z  TranslationCartesianOffset=[0.2243, -0.208, -0.283]  TranslationROffset=0  TranslationROffsetUnits=m  TranslationZOffset=0  TranslationZOffsetUnits=m  TranslationThetaOffset=0  TranslationThetaOffsetUnits=deg  RotationMethod=RotationSequence  RotationAngleUnits=deg  RotationStandardAxis=+Z  RotationAngle=0.0  RotationArbitraryAxis=[0 0 1]  FollAlignAxisA=+X  BaseAlignAxisA=+Y  FollAlignAxisB=+Y  BaseAlignAxisB=+Z  RotationSequenceAxes=BaseAxes  RotationSequence=XYZ  RotationSequenceAngles=[0, 0, 0]  RotationSequenceAnglesUnits=rad  RotationMatrix=[1 0 0; 0 1 0; 0 0 1]
  Visual : sm_lib/Body Elements/File Solid  ExtGeomFileName=C:\Users\河明山\Desktop\毕业设计\下肢\meshes\Back_Base_Link.STL  UnitType=Custom  ExtGeomFileUnits=m  StepReaderType=HEX  ExportConvexHullGeometry=off  InertiaType=Custom  Mass=0  MassUnits=kg  CenterOfMass=[0, 0, 0]  CenterOfMassUnits=m  MomentsOfInertia=[0, 0, 0]  MomentsOfInertiaUnits=kg*m^2  ProductsOfInertia=[0, 0, 0]  ProductsOfInertiaUnits=kg*m^2  BasedOnType=DensityFromFile  Density=1000  DensityUnits=kg/m^3  DoExposeReferenceFrame=on  SerializedFrames=<Frames/>  GraphicType=FromGeometry  MarkerShape=Sphere  MarkerSize=10  GraphicVisPropType=SimpleVisualProperties  GraphicDiffuseColor=[0.898039215686275, 0.917647058823529, 0.929411764705882]  GraphicSpecularColor=[0.5 0.5 0.5 1.0]  GraphicAmbientColor=[0.15 0.15 0.15 1.0]  GraphicEmissiveColor=[0.0 0.0 0.0 1.0]  GraphicShininess=75  GraphicOpacity=1
  VisualOriginTransform : sm_lib/Frames and Transforms/Rigid Transform  TranslationMethod=Cartesian  TranslationStandardOffset=0  TranslationLengthUnit=m  TranslationStandardAxis=+Z  TranslationCartesianOffset=[0, 0, 0]  TranslationROffset=0  TranslationROffsetUnits=m  TranslationZOffset=0  TranslationZOffsetUnits=m  TranslationThetaOffset=0  TranslationThetaOffsetUnits=deg  RotationMethod=RotationSequence  RotationAngleUnits=deg  RotationStandardAxis=+Z  RotationAngle=0.0  RotationArbitraryAxis=[0 0 1]  FollAlignAxisA=+X  BaseAlignAxisA=+Y  FollAlignAxisB=+Y  BaseAlignAxisB=+Z  RotationSequenceAxes=BaseAxes  RotationSequence=XYZ  RotationSequenceAngles=[0, 0, 0]  RotationSequenceAnglesUnits=rad  RotationMatrix=[1 0 0; 0 1 0; 0 0 1]
  F : PMIOPort  Side=Left
  F2 : PMIOPort  Port=2  Side=Right
  F1 : PMIOPort  Port=3  Side=Right
  connections:
  Inertia/RConn1 -- InertiaOriginTransform/RConn1
  Left_Hip_Joint_AxisTransform/RConn1 -- F1/RConn1
  Left_Hip_Joint_AxisTransform/LConn1 -- Left_Hip_Joint_OriginTransform/RConn1
  Left_Hip_Joint_OriginTransform/LConn1 -- InertiaOriginTransform/LConn1 -- ReferenceFrame/RConn1 -- F/RConn1 -- VisualOriginTransform/LConn1 -- Right_Hip_Joint_OriginTransform/LConn1
  Right_Hip_Joint_AxisTransform/RConn1 -- F2/RConn1
  Right_Hip_Joint_AxisTransform/LConn1 -- Right_Hip_Joint_OriginTransform/RConn1
  Visual/RConn1 -- VisualOriginTransform/RConn1

== system PID_Position_Control/Robot/Robot/robot/Left_Ankle_Link ==
  Inertia : sm_lib/Body Elements/Inertia  InertiaType=Custom  Mass=1.19036450922831  MassUnits=kg  CenterOfMass=[0, 0, 0]  CenterOfMassUnits=m  MomentsOfInertia=[0.00153091818368035, 0.0064801204508979, 0.00598779799807743]  MomentsOfInertiaUnits=kg*m^2  ProductsOfInertia=[-7.19796708189506e-06, 6.995899556434e-05, -6.61160505400838e-06]  ProductsOfInertiaUnits=kg*m^2  GraphicType=None  MarkerShape=Inertia  MarkerSize=20  GraphicVisPropType=SimpleVisualProperties  GraphicDiffuseColor=[0.5 0.5 0.5]  GraphicSpecularColor=[0.5 0.5 0.5 1.0]  GraphicAmbientColor=[0.15 0.15 0.15 1.0]  GraphicEmissiveColor=[0.0 0.0 0.0 1.0]  GraphicShininess=75  GraphicOpacity=1.0
  InertiaOriginTransform : sm_lib/Frames and Transforms/Rigid Transform  TranslationMethod=Cartesian  TranslationStandardOffset=0  TranslationLengthUnit=m  TranslationStandardAxis=+Z  TranslationCartesianOffset=[0.0464300413622986, 0.07679180433861869, -0.0192031324458123]  TranslationROffset=0  TranslationROffsetUnits=m  TranslationZOffset=0  TranslationZOffsetUnits=m  TranslationThetaOffset=0  TranslationThetaOffsetUnits=deg  RotationMethod=RotationSequence  RotationAngleUnits=deg  RotationStandardAxis=+Z  RotationAngle=0.0  RotationArbitraryAxis=[0 0 1]  FollAlignAxisA=+X  BaseAlignAxisA=+Y  FollAlignAxisB=+Y  BaseAlignAxisB=+Z  RotationSequenceAxes=BaseAxes  RotationSequence=XYZ  RotationSequenceAngles=[0, 0, 0]  RotationSequenceAnglesUnits=rad  RotationMatrix=[1 0 0; 0 1 0; 0 0 1]
  Left_Ankle_Joint_AxisInvTransform : sm_lib/Frames and Transforms/Rigid Transform  TranslationMethod=Cartesian  TranslationStandardOffset=0  TranslationLengthUnit=m  TranslationStandardAxis=+Z  TranslationCartesianOffset=[0, 0, 0]  TranslationROffset=0  TranslationROffsetUnits=m  TranslationZOffset=0  TranslationZOffsetUnits=m  TranslationThetaOffset=0  TranslationThetaOffsetUnits=deg  RotationMethod=ArbitraryAxis  RotationAngleUnits=rad  RotationStandardAxis=+Z  RotationAngle=0  RotationArbitraryAxis=[1, 0, 0]  FollAlignAxisA=+X  BaseAlignAxisA=+Y  FollAlignAxisB=+Y  BaseAlignAxisB=+Z  RotationSequenceAxes=FollowerAxes  RotationSequence=XYX  RotationSequenceAngles=[0 0 0]  RotationSequenceAnglesUnits=deg  RotationMatrix=[1 0 0; 0 1 0; 0 0 1]
  ReferenceFrame : sm_lib/Frames and Transforms/Reference Frame
  Visual : sm_lib/Body Elements/File Solid  ExtGeomFileName=C:\Users\河明山\Desktop\毕业设计\下肢\meshes\Left_Ankle_Link.STL  UnitType=Custom  ExtGeomFileUnits=m  StepReaderType=HEX  ExportConvexHullGeometry=off  InertiaType=Custom  Mass=0  MassUnits=kg  CenterOfMass=[0, 0, 0]  CenterOfMassUnits=m  MomentsOfInertia=[0, 0, 0]  MomentsOfInertiaUnits=kg*m^2  ProductsOfInertia=[0, 0, 0]  ProductsOfInertiaUnits=kg*m^2  BasedOnType=DensityFromFile  Density=1000  DensityUnits=kg/m^3  DoExposeReferenceFrame=on  SerializedFrames=<Frames/>  GraphicType=FromGeometry  MarkerShape=Sphere  MarkerSize=10  GraphicVisPropType=SimpleVisualProperties  GraphicDiffuseColor=[0.898039215686275, 0.917647058823529, 0.929411764705882]  GraphicSpecularColor=[0.5 0.5 0.5 1.0]  GraphicAmbientColor=[0.15 0.15 0.15 1.0]  GraphicEmissiveColor=[0.0 0.0 0.0 1.0]  GraphicShininess=75  GraphicOpacity=1
  VisualOriginTransform : sm_lib/Frames and Transforms/Rigid Transform  TranslationMethod=Cartesian  TranslationStandardOffset=0  TranslationLengthUnit=m  TranslationStandardAxis=+Z  TranslationCartesianOffset=[0, 0, 0]  TranslationROffset=0  TranslationROffsetUnits=m  TranslationZOffset=0  TranslationZOffsetUnits=m  TranslationThetaOffset=0  TranslationThetaOffsetUnits=deg  RotationMethod=RotationSequence  RotationAngleUnits=deg  RotationStandardAxis=+Z  RotationAngle=0.0  RotationArbitraryAxis=[0 0 1]  FollAlignAxisA=+X  BaseAlignAxisA=+Y  FollAlignAxisB=+Y  BaseAlignAxisB=+Z  RotationSequenceAxes=BaseAxes  RotationSequence=XYZ  RotationSequenceAngles=[0, 0, 0]  RotationSequenceAnglesUnits=rad  RotationMatrix=[1 0 0; 0 1 0; 0 0 1]
  F : PMIOPort  Side=Left
  connections:
  Inertia/RConn1 -- InertiaOriginTransform/RConn1
  Left_Ankle_Joint_AxisInvTransform/RConn1 -- F/RConn1
  Left_Ankle_Joint_AxisInvTransform/LConn1 -- InertiaOriginTransform/LConn1 -- ReferenceFrame/RConn1 -- VisualOriginTransform/LConn1
  Visual/RConn1 -- VisualOriginTransform/RConn1
